simulink model "TrabalhoFuzzyNivel_v02"  (R2014b)
settings: Solver=ode1  StartTime=0.0  StopTime=1696  FixedStep=0.1  RelTol=1e-3  EnableMultiTasking=on
InitFcn:
  | R1
  | R2
  | C1
  | C2
  | Q_max
  | T
  | H1_max
  | H2_max
values from neighbouring files (symbols this model uses):
  C1 = pi*0.35^2    (= 0.384845100065)    [TrabalhoFuzzy.m]
  C2 = beta*C1    (= 0.153938040026)    [TrabalhoFuzzy.m]
  Q_max = 0.0083    [TrabalhoFuzzy.m]
  R1 = 0.4*R2    (= 192.771084337)    [TrabalhoFuzzy.m]
  R2 = 4/Q_max    (= 481.927710843)    [TrabalhoFuzzy.m]
libraries: fuzblock x2
settings Model: Creator=Thiago Werneck  LastModifiedBy=Thiago Werneck
settings SolverCC: AutoInsertRateTranBlk=on
settings OptimizationCC: UseDivisionForNetSlopeComputation=off  SimCompilerOptimization=off
settings DebuggingCC: FcnCallInpInsideContextMsg=error  FrameProcessingCompatibilityMsg=error  SFExecutionAtInitializationDiag=none
settings HardwareCC: ProdBitPerSizeT=32  ProdBitPerPtrDiffT=32
settings RTWCC: RTWCompilerOptimization=off
settings CodeAppCC: StateflowObjectComments=on
settings ConfigComp: CovMetricSettings=dw  CovHtmlReporting=on  CovSaveCumulativeToWorkspaceVar=on  CovSaveSingleToWorkspaceVar=on  CovExternalEMLEnable=off  CovSFcnEnable=off

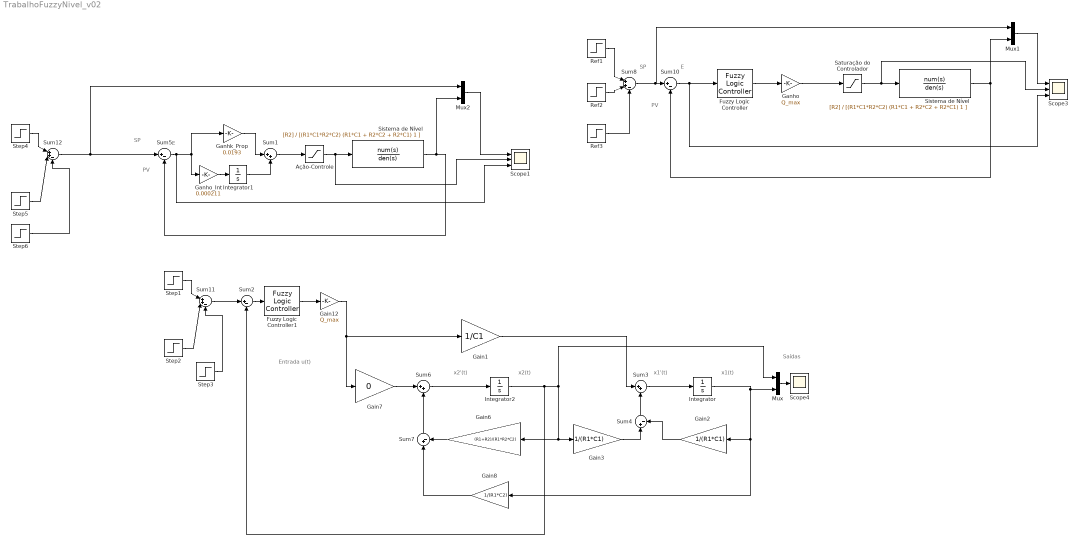
== system TrabalhoFuzzyNivel_v02 ==
  note: SP
  note: Saídas
  note: x1'(t)
  note: Entrada u(t)
  note: x1(t)
  note: x2'(t)
  note: x2(t)
  note: PV
  note: E
  note: SP
  note: E
  note: PV
  Ação-Controle : Saturate  UpperLimit=Q_max  LowerLimit=0
  Fuzzy Logic Controller : fuzblock/Fuzzy Logic  Controller  fis='TankLevelControl17.fis'
  Fuzzy Logic Controller1 : fuzblock/Fuzzy Logic  Controller  fis='TankLevelControl17.fis'
  Gain1 : Gain  Gain=1/C1
  Gain12 : Gain  Gain=Q_max
  Gain2 : Gain  Gain=1/(R1*C1)
  Gain3 : Gain  Gain=1/(R1*C1)
  Gain6 : Gain  Gain=(R1+R2)/(R1*R2*C2)
  Gain7 : Gain  Gain=0
  Gain8 : Gain  Gain=1/(R1*C2)
  "Ganhk_Prop " : Gain  Gain=0.0193
  "Ganho " : Gain  Gain=Q_max
  "Ganho_Int " : Gain  Gain=0.000211
  Integrator : Integrator
  Integrator1 : Integrator  UpperSaturationLimit=Q_max  LowerSaturationLimit=0
  Integrator2 : Integrator
  Mux : Mux  Inputs=2
  Mux1 : Mux  Inputs=2
  Mux2 : Mux  Inputs=2
  "Ref1 " : Step  Time=2000  After=1.2  SampleTime=1
  Ref2 : Step  Time=100  After=1.2  SampleTime=1
  Ref3 : Step  Time=1000  After=0.6  SampleTime=1
  Saturação do Controlador : Saturate  UpperLimit=Q_max  LowerLimit=0
  Scope1 : Scope  NumInputPorts=3
      settings: TimeRange=3770  YMin=-5~-5~-5  YMax=5~5~5  SaveName=PI_Control  MaxDataPoints=6000
  Scope3 : Scope  NumInputPorts=3
      settings: TimeRange=3770  YMin=0.5~0~-0.2  YMax=2~0.008~1.4  SaveName=FuzzyLogic
  Scope4 : Scope
      settings: ShowLegends=on  TimeRange=3770  SaveName=saida  Decimation=12
  Sistema de Nível : TransferFcn  Numerator=[R2]  Denominator=[(R1*C1*R2*C2) (R1*C1 + R2*C2 + R2*C1) 1 ]
  "Sistema de Nível " : TransferFcn  Numerator=[R2]  Denominator=[(R1*C1*R2*C2) (R1*C1 + R2*C2 + R2*C1) 1 ]
  Step1 : Step  Time=4000  After=1.2  SampleTime=1
  Step2 : Step  Time=1000  After=1.2  SampleTime=1
  Step3 : Step  Time=2000  After=0.6  SampleTime=1
  Step4 : Step  Time=2000  After=1.2  SampleTime=1
  Step5 : Step  Time=100  After=1.2  SampleTime=1
  Step6 : Step  Time=1000  After=0.6  SampleTime=1
  Sum1 : Sum  Inputs=|++
  Sum{2,4..5,7,10} (5 alike) : Sum  Inputs=|+-
  Sum11 : Sum  Inputs=|++-
  Sum12 : Sum  Inputs=|++-
  Sum3 : Sum  Inputs=|++
  Sum6 : Sum  Inputs=|++
  Sum8 : Sum  Inputs=|++-
  wires:
  Sistema de Nível/1 -> Mux2/2, Sum5/2
  Ação-Controle/1 -> Scope1/2, Sistema de Nível/1
  Sum5/1 -> Scope1/3, "Ganhk_Prop "/1, "Ganho_Int "/1
  "Ganho_Int "/1 -> Integrator1/1
  "Ganhk_Prop "/1 -> Sum1/1
  Integrator1/1 -> Sum1/2
  Sum1/1 -> Ação-Controle/1
  Gain1/1 -> Sum3/1
  Sum3/1 -> Integrator/1
  Integrator/1 -> Mux/2, Gain8/1, Gain2/1
  Gain2/1 -> Sum4/2
  Gain7/1 -> Sum6/1
  Sum6/1 -> Integrator2/1
  Integrator2/1 -> Sum2/2, Mux/1, Gain3/1, Gain6/1
  Gain6/1 -> Sum7/2
  Sum7/1 -> Sum6/2
  Gain8/1 -> Sum7/1
  Gain3/1 -> Sum4/1
  Sum4/1 -> Sum3/2
  Mux/1 -> Scope4/1
  Saturação do Controlador/1 -> Scope3/2, "Sistema de Nível "/1
  "Ref1 "/1 -> Sum8/1
  Sum8/1 -> Mux1/1, Sum10/1
  Ref2/1 -> Sum8/2
  Sum10/1 -> Fuzzy Logic Controller/1, Scope3/3
  Fuzzy Logic Controller/1 -> "Ganho "/1
  "Ganho "/1 -> Saturação do Controlador/1
  Ref3/1 -> Sum8/3
  "Sistema de Nível "/1 -> Sum10/2, Mux1/2
  Fuzzy Logic Controller1/1 -> Gain12/1
  Gain12/1 -> Gain1/1, Gain7/1
  Sum2/1 -> Fuzzy Logic Controller1/1
  Step1/1 -> Sum11/1
  Sum11/1 -> Sum2/1
  Step2/1 -> Sum11/2
  Step3/1 -> Sum11/3
  Mux1/1 -> Scope3/1
  Step4/1 -> Sum12/1
  Step5/1 -> Sum12/2
  Step6/1 -> Sum12/3
  Sum12/1 -> Mux2/1, Sum5/1
  Mux2/1 -> Scope1/1
